simulink model "transmitacja"  (R2019b)
settings: Solver=VariableStepAuto  StartTime=0.0  StopTime=10.0  RelTol=1e-3
values from neighbouring files (symbols this model uses):
  d_Tz = 0    [WyznaczenieStatycznych.m]    (also in Wyznaczenie_K.m; onlyfp.m; state.m; transmitancja.m)
  d_Tzew = 0    [WyznaczenieStatycznych.m]    (also in Wyznaczenie_K.m; onlyfp.m; state.m = 3; transmitancja.m = 3)
  L11 = [Cvp*c, c*b]    [transmitancja.m]
  L12 = [Kw*Cvp, Kw*b+K1*Kp]    [transmitancja.m]
  L21 = [K1*c]    [transmitancja.m]
  L22 = [Cvw*Kp, a*Kp+Kw*K1]    [transmitancja.m]
  M = [Cvw*Cvp,(Cvw*b+Cvp*a),a*b-K1^2]    [transmitancja.m]
  t_skok = 100    [WyznaczenieStatycznych.m]    (also in Wyznaczenie_K.m = 500; onlyfp.m = 500; state.m = 500; transmitancja.m = 500)
  Tp0 = TpN    (= 18)    [WyznaczenieStatycznych.m]    (also in Wyznaczenie_K.m = Y(2); onlyfp.m = Y(2); state.m = Y(2); transmitancja.m = Y(2))
  Twew0 = TwewN    (= 22)    [WyznaczenieStatycznych.m]    (also in Wyznaczenie_K.m = Y(1); onlyfp.m = Y(1); state.m = Y(1); transmitancja.m = Y(1))
settings Model: Creator=Mariusz  LastModifiedBy=Mariusz

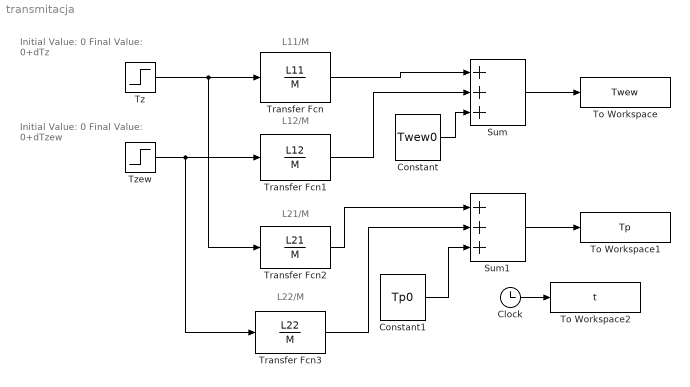
== system transmitacja ==
  note: L22/M
  note: L21/M
  note: L12/M
  note: L11/M
  note: Initial Value: 0
      | Final Value: 0+dTz
  note: Initial Value: 0
      | Final Value: 0+dTzew
  Clock : Clock
  Constant : Constant  Value=Twew0
  Constant1 : Constant  Value=Tp0
  Sum : Sum  Inputs=+++
  Sum1 : Sum  Inputs=+++
  To Workspace : ToWorkspace  VariableName=Twew  SampleTime=-1
  To Workspace1 : ToWorkspace  VariableName=Tp  SampleTime=-1
  To Workspace2 : ToWorkspace  VariableName=t  SampleTime=-1
  Transfer Fcn : TransferFcn  Numerator=L11  Denominator=M
  Transfer Fcn1 : TransferFcn  Numerator=L12  Denominator=M
  Transfer Fcn2 : TransferFcn  Numerator=L21  Denominator=M
  Transfer Fcn3 : TransferFcn  Numerator=L22  Denominator=M
  Tz : Step  Time=t_skok  After=0 + d_Tz  SampleTime=0
  Tzew : Step  Time=t_skok  After=0 + d_Tzew  SampleTime=0
  wires:
  Tz/1 -> Transfer Fcn2/1, Transfer Fcn/1
  Transfer Fcn/1 -> Sum/1
  Transfer Fcn1/1 -> Sum/2
  Tzew/1 -> Transfer Fcn3/1, Transfer Fcn1/1
  Transfer Fcn3/1 -> Sum1/2
  Transfer Fcn2/1 -> Sum1/1
  Constant/1 -> Sum/3
  Constant1/1 -> Sum1/3
  Clock/1 -> To Workspace2/1
  Sum/1 -> To Workspace/1
  Sum1/1 -> To Workspace1/1
